simulink subsystem "Logica_bateria"  (R2023b)
settings: Solver=VariableStepAuto  StartTime=0.0  StopTime=10.0  RelTol=1e-3
settings Model: Creator=Usuario_UMA  LastModifiedBy=Usuario_UMA

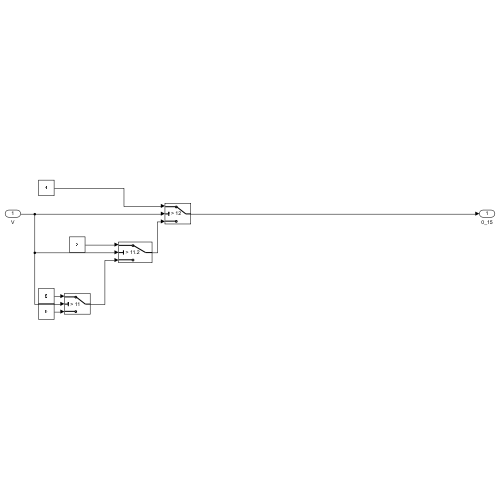
[thumbnail: Simulink's stored preview of the top-level diagram]
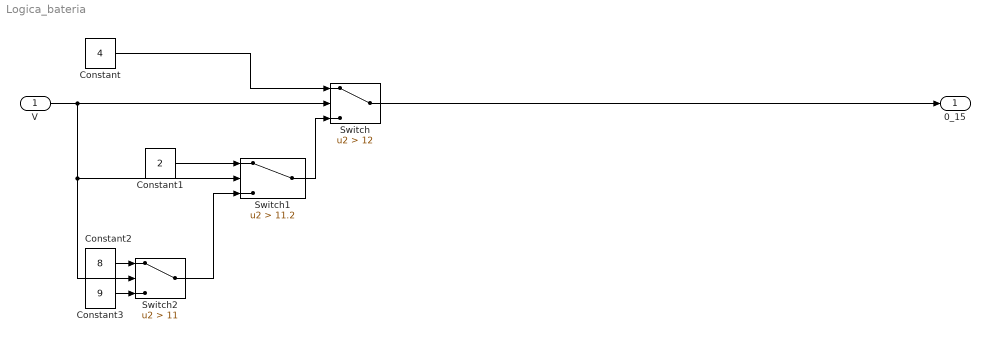
== system Logica_bateria ==
  V : Inport
  Constant : Constant  Value=4
  Constant1 : Constant  Value=2
  Constant2 : Constant  Value=8
  Constant3 : Constant  Value=9
  Switch : Switch  Criteria=u2 > Threshold  Threshold=12  SaturateOnIntegerOverflow=off  InputSameDT=off
  Switch1 : Switch  Criteria=u2 > Threshold  Threshold=11.2  SaturateOnIntegerOverflow=off  InputSameDT=off
  Switch2 : Switch  Criteria=u2 > Threshold  Threshold=11  SaturateOnIntegerOverflow=off  InputSameDT=off
  0_15 : Outport
  wires:
  V/1 -> Switch2/2, Switch1/2, Switch/2
  Constant/1 -> Switch/1
  Switch/1 -> 0_15/1
  Switch1/1 -> Switch/3
  Switch2/1 -> Switch1/3
  Constant1/1 -> Switch1/1
  Constant2/1 -> Switch2/1
  Constant3/1 -> Switch2/3
